simulink model "test"  (Simulink 8.5)
settings: Solver=ode45  StartTime=0.0  StopTime=100000.0  RelTol=1e-3
model workspace: external: MATLAB Code (data not in the file)
libraries: commdigbbndpm3 x2, commchan3 x1, commsink2 x1, commrflib2 x1, commrandsrc2 x1
settings Model: Creator=francisco  LastModifiedBy=francisco
settings DataIOCC: SignalLoggingSaveFormat=Dataset
settings OptimizationCC: ExpressionDepthLimit=128
settings DebuggingCC: UnderspecifiedInitializationDetection=Simplified  MergeDetectMultiDrivingBlocksExec=error  FcnCallInpInsideContextMsg=EnableAllAsError  StateNameClashWarn=none
settings GRTTargetCC: CombineOutputUpdateFcns=on  GRTInterface=off

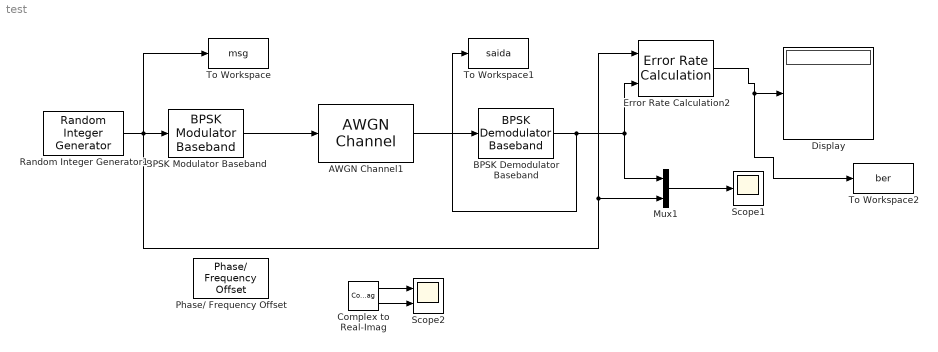
== system test ==
  AWGN Channel1 : commchan3/AWGN Channel  InputProcessing=Columns as channels (frame based)  seed=67  noiseMode="Signal to noise ratio  (Eb/No)"  EbNodB=EbNo  EsNodB=10  SNRdB=10  bitsPerSym=1  Ps=1  Tsym=1  variance=1
  BPSK Demodulator Baseband : commdigbbndpm3/BPSK Demodulator Baseband  Ph=0  DecType=Hard decision  VarSource=Dialog  Variance=1  outDtype=Inherit via internal rule  derotateFactorWordLen=16
  BPSK Modulator Baseband : commdigbbndpm3/BPSK Modulator Baseband  Ph=0  outDtype=double  outWordLen=16  outUDDataType=sfix(16)  outFracLenMode=Best precision  outFracLen=15
  Complex to Real-Imag : ComplexToRealImag
  Display : Display
  Error Rate Calculation2 : commsink2/Error Rate Calculation  N=0  st_delay=0  cp_mode=Entire frame  subframe=[]  PMode=Port  WsName=ErrorVec  RsMode2=off  stop=off  numErr=100  maxBits=1e6
  Mux1 : Mux  Inputs=2
  Phase/ Frequency Offset : commrflib2/Phase// Frequency Offset  phaseOffset=10  freqPort=off  freqOffset=0
  Random Integer Generator1 : commrandsrc2/Random Integer Generator  RequirementInfo="{}  %GIDa_f806ea20_e19a_4035_a8ac_7d6336cc0989"  mul=2  seed=37  Ts=1  frameBased=off  sampPerFrame=1  orient=off  outDataType=double
  Scope1 : Scope
      settings: SaveName=ScopeData2  Decimation=100
  Scope2 : Scope  NumInputPorts=2
      settings: YMin=-5~-5  YMax=5~5
  To Workspace : ToWorkspace  VariableName=msg  SaveFormat=Timeseries  SampleTime=-1
  To Workspace1 : ToWorkspace  VariableName=saida  SaveFormat=Timeseries  SampleTime=-1
  To Workspace2 : ToWorkspace  VariableName=ber  SampleTime=-1
      settings: MaxDataPoints=2  Save2DSignal=2-D array (concatenate along first dimension)
  wires:
  Random Integer Generator1/1 -> BPSK Modulator Baseband/1, To Workspace/1, Error Rate Calculation2/1, Mux1/2
  BPSK Demodulator Baseband/1 -> To Workspace1/1, Error Rate Calculation2/2, Mux1/1
  Mux1/1 -> Scope1/1
  Complex to Real-Imag/1 -> Scope2/1
  Complex to Real-Imag/2 -> Scope2/2
  BPSK Modulator Baseband/1 -> AWGN Channel1/1
  Error Rate Calculation2/1 -> To Workspace2/1, Display/1
  AWGN Channel1/1 -> BPSK Demodulator Baseband/1
